simulink model "CA3_model_velocity"  (R2023b)
settings: Solver=VariableStepAuto  StartTime=0.0  StopTime=10  RelTol=1e-3
values from neighbouring files (symbols this model uses):
  b = [0;0;1]    [CA3_velocity_param.m]
  C = 1    [CA3_velocity_param.m]
  Gamma = [1 0 0; 0 1 0; 0 0 1]    [CA3_velocity_param.m]
  gamma = 1    [CA3_velocity_param.m]
  K = 6.2    [CA3_velocity_param.m]
  k_w = mdl2.Coefficients{1,1}    [CA3_velocity_param.m]
  P = lyap(Am', Q)    [CA3_velocity_param.m]
  tau = 0.25    [CA3_velocity_param.m]
  w = 10    [CA3_velocity_param.m]
settings Model: Creator=jiang  LastModifiedBy=99551
settings SolverCC: ZeroCrossAlgorithm=Adaptive
settings DebuggingCC: IgnoredZcDiagnostic=none  UnconnectedInputMsg=warning  UnconnectedOutputMsg=warning  UnconnectedLineMsg=warning
settings ModelReferenceCC: EnableRefExpFcnMdlSchedulingChecks=on
settings RTWCC: DLArmComputeVersion=19.05

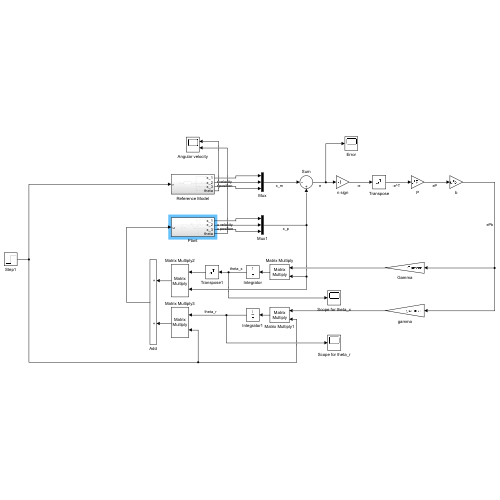
[thumbnail: Simulink's stored preview of the top-level diagram]
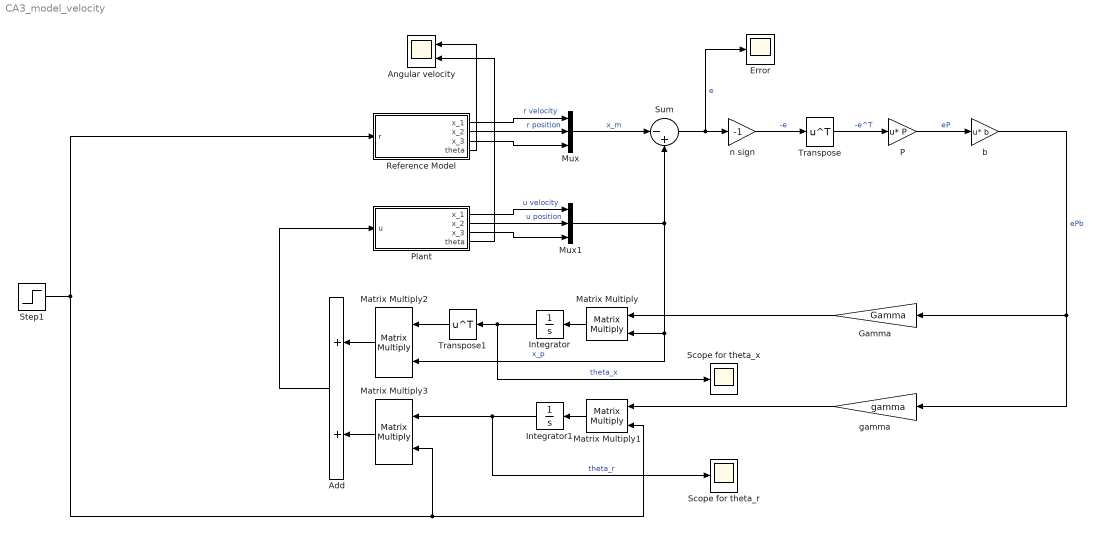
== system CA3_model_velocity ==
  Add : Sum
  Angular velocity : Scope  NumInputPorts=2
  Error : Scope
  Gamma : Gain  Gain=Gamma
  Integrator : Integrator
  Integrator1 : Integrator
  Matrix Multiply{,1..3} (4 alike) : Product  Multiplication=Matrix(*)
  Mux : Mux  Inputs=3
  Mux1 : Mux  Inputs=3
  P : Gain  Gain=P  Multiplication=Matrix(u*K)
  Plant : Subsystem
  Reference Model : Subsystem
  Scope for theta_r : Scope
  Scope for theta_x : Scope
  Step1 : Step  SampleTime=0
  Sum : Sum  Inputs=|-+
  Transpose : Math  Operator=transpose
  Transpose1 : Math  Operator=transpose
  b : Gain  Gain=b  Multiplication=Matrix(u*K)
  gamma : Gain  Gain=gamma
  n sign : Gain  Gain=-1
  wires:
  Mux/1 -> Sum/1  "x_m"
  Mux1/1 -> Matrix Multiply2/2, Matrix Multiply/2, Sum/2  "x_p"
  Sum/1 -> Error/1, n sign/1  "e"
  n sign/1 -> Transpose/1  "-e"
  Transpose/1 -> P/1  "-e^T"
  P/1 -> b/1  "eP"
  b/1 -> gamma/1, Gamma/1  "ePb"
  Gamma/1 -> Matrix Multiply/1
  gamma/1 -> Matrix Multiply1/1
  Matrix Multiply/1 -> Integrator/1
  Matrix Multiply1/1 -> Integrator1/1
  Integrator/1 -> Scope for theta_x/1, Transpose1/1  "theta_x"
  Transpose1/1 -> Matrix Multiply2/1
  Integrator1/1 -> Matrix Multiply3/1, Scope for theta_r/1  "theta_r"
  Matrix Multiply2/1 -> Add/1
  Matrix Multiply3/1 -> Add/2
  Reference Model/4(theta) -> Angular velocity/1
  Plant/4(theta) -> Angular velocity/2
  Add/1 -> Plant/1(u)
  Step1/1 -> Reference Model/1(r), Matrix Multiply3/2, Matrix Multiply1/2
  Reference Model/1(x_1) -> Mux/1  "r velocity"
  Reference Model/2(x_2) -> Mux/2  "r position"
  Reference Model/3(x_3) -> Mux/3
  Plant/1(x_1) -> Mux1/1  "u velocity"
  Plant/2(x_2) -> Mux1/2  "u position"
  Plant/3(x_3) -> Mux1/3

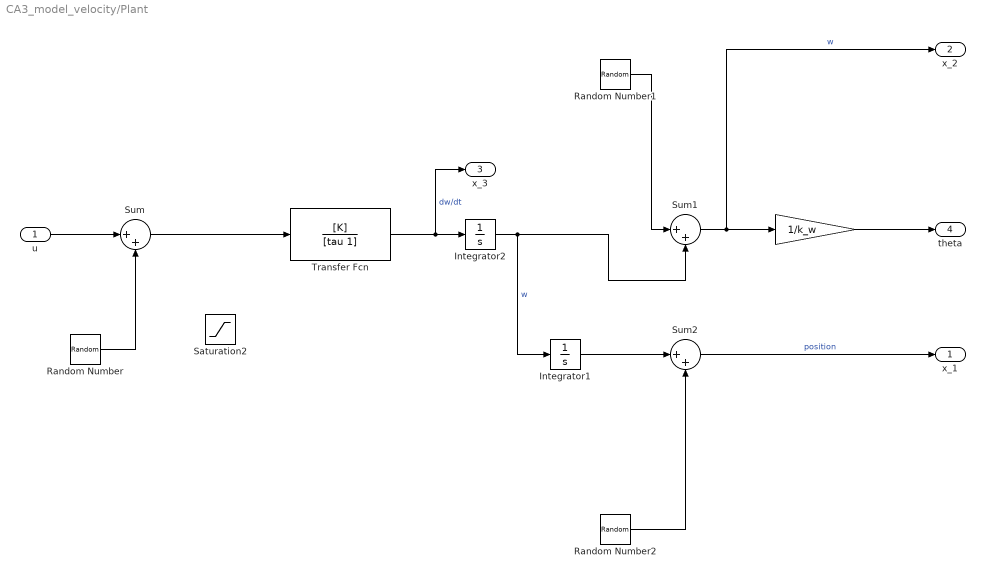
== system CA3_model_velocity/Plant ==
  u : Inport
  " " : Gain  Gain=1/k_w
  Integrator1 : Integrator
  Integrator2 : Integrator
  Random Number : RandomNumber  Variance=0.1  SampleTime=0.01
  Random Number1 : RandomNumber  Variance=0.0001  SampleTime=0.01
  Random Number2 : RandomNumber  Variance=0.0001  SampleTime=0.01
  Saturation2 : Saturate  UpperLimit=5  LowerLimit=-5
  Sum : Sum  Inputs=|++
  Sum1 : Sum  Inputs=|++
  Sum2 : Sum  Inputs=|++
  Transfer Fcn : TransferFcn  Numerator=[K]  Denominator=[tau 1]
  x_1 : Outport
  x_2 : Outport  Port=2
  x_3 : Outport  Port=3
  theta : Outport  Port=4
  wires:
  u/1 -> Sum/1
  Transfer Fcn/1 -> x_3/1, Integrator2/1  "dw/dt"
  Sum1/1 -> x_2/1, " "/1  "w"
  Sum2/1 -> x_1/1  "position"
  " "/1 -> theta/1
  Integrator1/1 -> Sum2/1
  Integrator2/1 -> Sum1/2, Integrator1/1  "w"
  Random Number2/1 -> Sum2/2
  Random Number/1 -> Sum/2
  Sum/1 -> Transfer Fcn/1
  Random Number1/1 -> Sum1/1

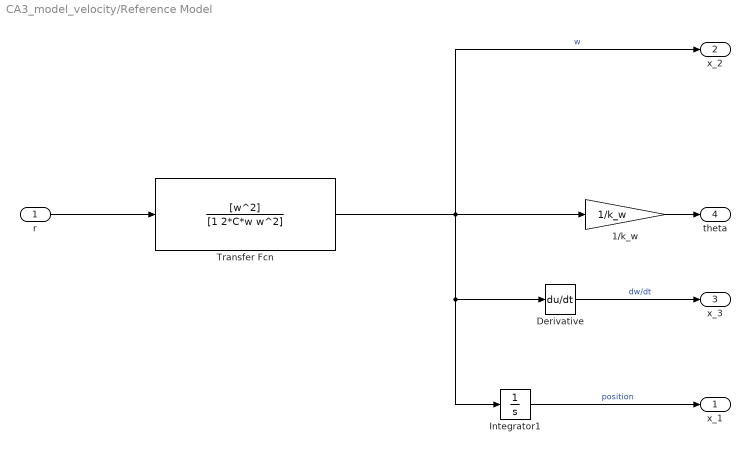
== system CA3_model_velocity/Reference Model ==
  r : Inport
  1/k_w : Gain  Gain=1/k_w
  Derivative : Derivative
  Integrator1 : Integrator
  Transfer Fcn : TransferFcn  Numerator=[w^2]  Denominator=[1 2*C*w w^2]
  x_1 : Outport
  x_2 : Outport  Port=2
  x_3 : Outport  Port=3
  theta : Outport  Port=4
  wires:
  r/1 -> Transfer Fcn/1
  Transfer Fcn/1 -> x_2/1, 1/k_w/1, Derivative/1, Integrator1/1  "w"
  1/k_w/1 -> theta/1
  Integrator1/1 -> x_1/1  "position"
  Derivative/1 -> x_3/1  "dw/dt"
